simulink model "conveyor_belt_system_models_in_simulink"  (R2023a)
settings: Solver=VariableStepAuto  StartTime=0.0  StopTime=120  RelTol=1e-3
undefined symbols (not defined in the file): b, Fv, G, J, K1, K2, K3, Kphi, L, Mc, R, R_pully
libraries: slpidlib x1
settings Model: Creator=ARABI  LastModifiedBy=ARABI

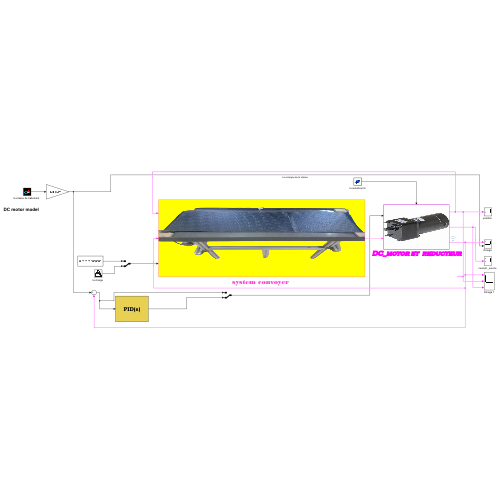
[thumbnail: Simulink's stored preview of the top-level diagram]
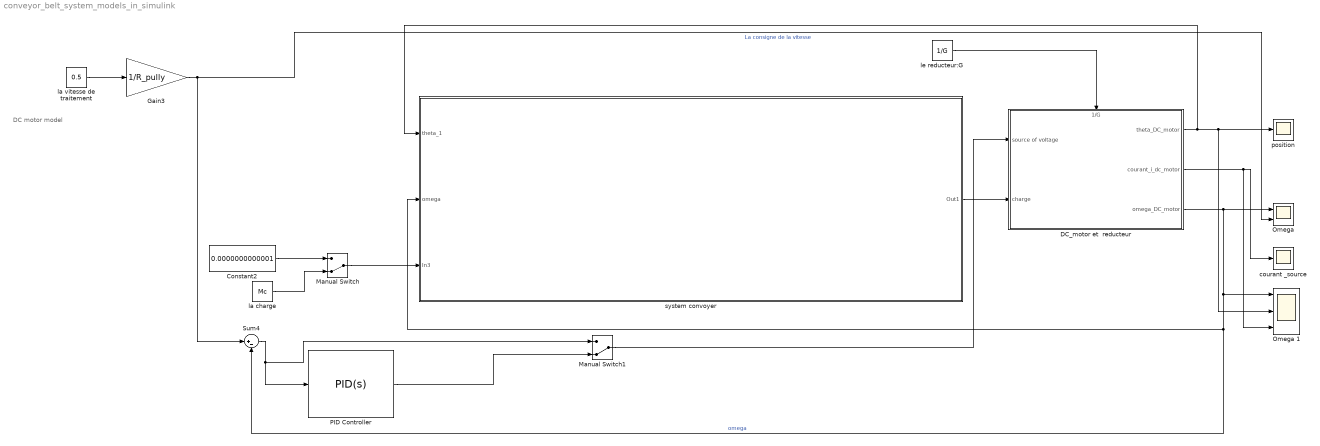
== system conveyor_belt_system_models_in_simulink ==
  note: DC motor model
  Constant2 : Constant  Value=0.0000000000001
  DC_motor et  reducteur : Subsystem
      settings: PortSchema="{\"entries\":[{\"content\":{\"sides\":[{\"content\":{\"connectorIds\":[\"In1\",\"In2\"]},\"type\":\"ConnectorPlacement.EquallySpacedRectSide\",\"uuid\":\"26fbfc1a-56c7-4e56-9ac7-29104c9994d4\"},{\"content\":{\"connectorIds\":[\"Out1\",\"Out2\",\"Out3\"],\"side\":\"RIGHT\"},\"type\":\"ConnectorPlacement.EquallySpacedRectSide\",\"uuid\":\"e16094de-f307-4a64-93f4-279fc46fd241\"},{\"content\":{\"connectorIds\":[\"In3\"],\"side\":\"TOP\"},\"type\":\"ConnectorPlacement.EquallySpacedRectSide\",\"uuid\":\"6a3015f2-a4f9-4d11-9390-c80012a11723\"}]},\"type\":\"ConnectorPlacement.EquallySpacedConnector\",\"uuid\":\"83312b76-c8d9-4603-a222-ebea70a19c3f\"}],\"packageUris\":[\"http://schema.mathworks.com/mf0/Connector/R2020b\"],\"version\":\"1.0\"}"
      mask Display: image('OIP.jpeg'); % Use "Edit Image" on toolstrip to change.
  Gain3 : Gain  Gain=1/R_pully
  Manual Switch : ManualSwitch  CurrentSetting=0
  Manual Switch1 : ManualSwitch  CurrentSetting=0
  "Omega " : Scope  NumInputPorts=2
  Omega 1 : Scope  NumInputPorts=3
  PID Controller : slpidlib/PID Controller  Controller=PID  Form=Parallel  TimeDomain=Continuous-time  UseExternalTs=off  SampleTime=-1  IntegratorMethod=Forward Euler  FilterMethod=Forward Euler  ControllerParametersSource=internal  P=1  I=1  UseKiTs=off  D=0  N=100  UseFilter=on  TunerSelectOption=Transfer Function Based (PID Tuner App)  InitialConditionSource=internal  InitialConditionForIntegrator=0  InitialConditionForFilter=0  DifferentiatorICPrevScaledInput=0  ExternalReset=none  TrackingMode=off  Kt=1  LimitOutput=off  SatLimitsSource=internal  UpperSaturationLimit=inf  LowerSaturationLimit=-inf  LinearizeAsGain=on  AntiWindupMode=none  Kb=1  LimitIntegrator=off  UpperIntegratorSaturationLimit=inf  LowerIntegratorSaturationLimit=-inf  POutMin=[]  POutMax=[]  IOutMin=[]  IOutMax=[]  DOutMin=[]  DOutMax=[]  NOutMin=[]  NOutMax=[]  SumOutMin=[]  SumOutMax=[]  SaturationOutMin=[]  SaturationOutMax=[]  PParamMin=[]  PParamMax=[]  IParamMin=[]  IParamMax=[]  DParamMin=[]  DParamMax=[]  NParamMin=[]  NParamMax=[]  KbParamMin=[]  KbParamMax=[]  KtParamMin=[]  KtParamMax=[]  KbOutMin=[]  KbOutMax=[]  KtOutMin=[]  KtOutMax=[]  IntegratorOutMin=[]  IntegratorOutMax=[]  FilterOutMin=[]  FilterOutMax=[]  SumI1OutMin=[]  SumI1OutMax=[]  SumI2OutMin=[]  SumI2OutMax=[]  SumI3OutMin=[]  SumI3OutMax=[]  SumI4OutMin=[]  SumI4OutMax=[]  SumDOutMin=[]  SumDOutMax=[]  DifferentiatorOutMin=[]  DifferentiatorOutMax=[]  FilterDiffOutCoefMin=[]  FilterDiffOutCoefMax=[]  ReciprocalOutMin=[]  ReciprocalOutMax=[]  SumDenOutMin=[]  SumDenOutMax=[]  SumNumOutMin=[]  SumNumOutMax=[]  DivideOutMin=[]  DivideOutMax=[]  UdiffTsProdOutMin=[]  UdiffTsProdOutMax=[]  NTsProdOutMin=[]  NTsProdOutMax=[]  UintegralTsProdOutMin=[]  UintegralTsProdOutMax=[]  UngainTsProdOutMin=[]  UngainTsProdOutMax=[]  ClampingZeroOutDataTypeStr=Inherit: Inherit via back propagation  ClampingZeroOutMin=[]  ClampingZeroOutMax=[]  FilterDenConstantOutDataTypeStr=Inherit: Inherit via back propagation  FilterDenConstantOutMin=[]  FilterDenConstantOutMax=[]  PCopyOutDataTypeStr=Inherit: Inherit via back propagation  PCopyOutMin=[]  PCopyOutMax=[]  NCopyOutDataTypeStr=Inherit: Inherit via back propagation  NCopyOutMin=[]  NCopyOutMax=[]  IntegratorContinuousStateAttributes=''  IntegratorStateMustResolveToSignalObject=off  IntegratorRTWStateStorageClass=Auto  FilterContinuousStateAttributes=''  FilterStateMustResolveToSignalObject=off  FilterRTWStateStorageClass=Auto  ParallelPVariant=InternalParameters  IdealPVariant=Disabled  IVariant=InternalParameters  DVariant=InternalParameters  IntegratorVariant=Continuous  SatVariant=Disabled  AWVariant=Passthrough  PCopyVariant=Disabled  TRVariant=Disabled  FdbkBlocksVariant=Forward  IdealPFdbkVariant=Disabled  SatFdbkVariant=Disabled  DerivativeFilterVariant=ContFilter  NVariant=InternalParameters  NCopyVariant=Disabled  FilterICVariant=InternalICsFilter  IntegratorICVariant=InternalICs  ExternalResetVariant=Disabled  TRSumVariant=Passthrough  SumFdbkVariant=Disabled  SumVariant=Sum_PID  TsampFilterVariant=InternalTs  TsampNgainVariant=Passthrough  TsampIntegralVariant=Disabled_SignalSpec  ExternalSaturationOutDataTypeStr=Inherit: Same as second input
  Sum4 : Sum  Inputs=|+-
  "courant _source " : Scope
  "la charge " : Constant  Value=Mc
      mask Display: image('download (1).jpeg'); % Use "Edit Image" on toolstrip to change.
  "la vitesse de traitement  " : Constant  Value=0.5
      mask Display: image('download.jpeg'); % Use "Edit Image" on toolstrip to change.
  le reducteur:G : Constant  Value=1/G
      mask Display: image('Reductor-pendular-rossi.jpg'); % Use "Edit Image" on toolstrip to change.
  "position " : Scope
  "system convoyer " : Subsystem
      mask Display: image('$imagefile'); % Use "Edit Image" on toolstrip to change.
  wires:
  le reducteur:G/1 -> DC_motor et  reducteur/3(1/G)
  "la vitesse de traitement  "/1 -> Gain3/1
  Gain3/1 -> Sum4/1, "Omega "/2  "La consigne de la vitesse"
  "la charge "/1 -> Manual Switch/2
  Manual Switch/1 -> "system convoyer "/3(In3)
  Constant2/1 -> Manual Switch/1
  PID Controller/1 -> Manual Switch1/2
  Sum4/1 -> PID Controller/1, Manual Switch1/1
  "system convoyer "/1(Out1) -> DC_motor et  reducteur/2("charge ")
  Manual Switch1/1 -> DC_motor et  reducteur/1("source of voltage ")
  DC_motor et  reducteur/1(theta_DC_motor) -> "position "/1, Omega 1/2, "system convoyer "/1(theta_1)
  DC_motor et  reducteur/2(courant_i_dc_motor) -> Omega 1/3, "courant _source "/1
  DC_motor et  reducteur/3(omega_DC_motor) -> Sum4/2, "system convoyer "/2(omega), Omega 1/1, "Omega "/1  "omega"

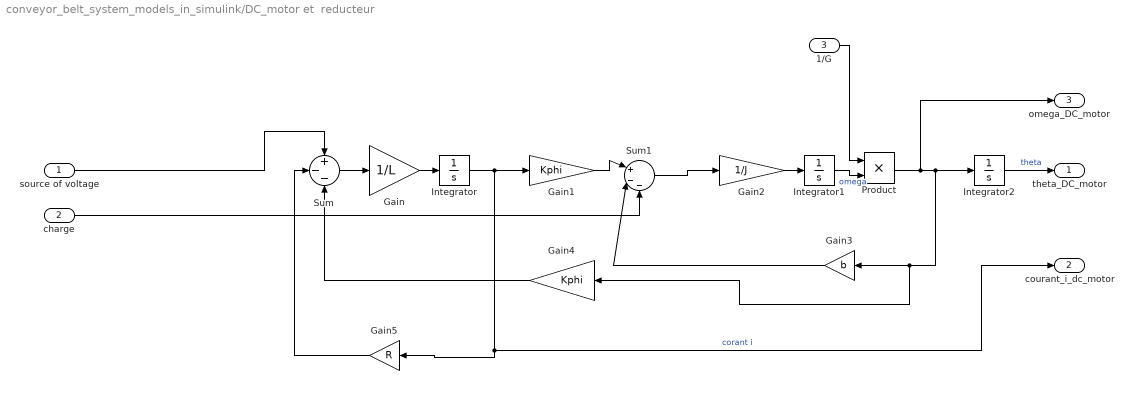
== system conveyor_belt_system_models_in_simulink/DC_motor et  reducteur ==
  "source of voltage " : Inport
  "charge " : Inport  Port=2
  1/G : Inport  Port=3
  Gain : Gain  Gain=1/L
  Gain1 : Gain  Gain=Kphi
  Gain2 : Gain  Gain=1/J
  Gain3 : Gain  Gain=b
  Gain4 : Gain  Gain=Kphi
  Gain5 : Gain  Gain=R
  Integrator : Integrator
  Integrator1 : Integrator
  Integrator2 : Integrator
  Product : Product
  Sum : Sum  Inputs=+--
  Sum1 : Sum  Inputs=|+--
  theta_DC_motor : Outport
  courant_i_dc_motor : Outport  Port=2
  omega_DC_motor : Outport  Port=3
  wires:
  "source of voltage "/1 -> Sum/1
  Sum/1 -> Gain/1
  Gain/1 -> Integrator/1
  Integrator/1 -> Gain5/1, courant_i_dc_motor/1, Gain1/1  "corant i"
  Gain1/1 -> Sum1/1
  Sum1/1 -> Gain2/1
  Gain2/1 -> Integrator1/1
  Integrator1/1 -> Product/2  "omega"
  Gain3/1 -> Sum1/2
  Gain4/1 -> Sum/3
  Gain5/1 -> Sum/2
  Integrator2/1 -> theta_DC_motor/1  "theta"
  "charge "/1 -> Sum1/3
  Product/1 -> omega_DC_motor/1, Integrator2/1, Gain4/1, Gain3/1
  1/G/1 -> Product/1

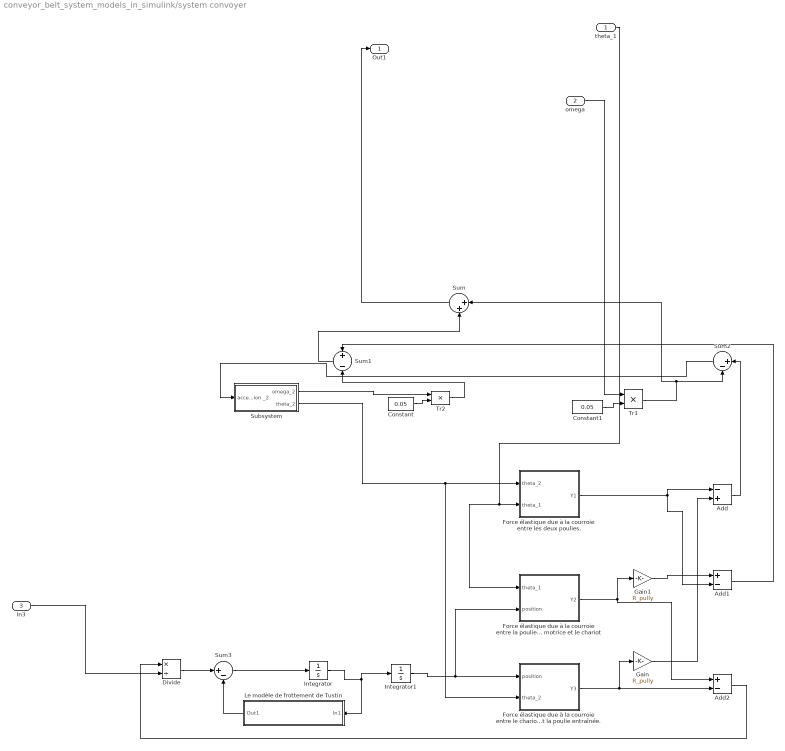
== system conveyor_belt_system_models_in_simulink/system convoyer  ==
  theta_1 : Inport
  omega : Inport  Port=2
  In3 : Inport  Port=3
  Add : Sum  Inputs=-+
  Add1 : Sum  Inputs=+-
  Add2 : Sum  Inputs=+-
  Constant : Constant  Value=0.05
  Constant1 : Constant  Value=0.05
  Divide : Product  Inputs=*/
  Force élastique due à la courroie entre la poulie motrice et le chariot : Subsystem
  Force élastique due à la courroie entre le chariot et la poulie entraînée. : Subsystem
  Force élastique due à la courroie entre les deux poulies. : Subsystem
  Gain : Gain  Gain=R_pully
  Gain1 : Gain  Gain=R_pully
  Integrator : Integrator
  Integrator1 : Integrator
  "Le modèle de frottement de Tustin " : Subsystem
  Subsystem : Subsystem
  Sum : Sum  Inputs=|++
  Sum1 : Sum  Inputs=+-
  Sum2 : Sum  Inputs=|+-
  Sum3 : Sum  Inputs=|+-
  Tr1 : Product
  Tr2 : Product
  Out1 : Outport
  wires:
  "Le modèle de frottement de Tustin "/1(Out1) -> Sum3/2
  theta_1/1 -> Force élastique due à la courroie entre la poulie motrice et le chariot/1(theta_1), Force élastique due à la courroie entre les deux poulies./2(theta_1)
  Force élastique due à la courroie entre le chariot et la poulie entraînée./1(Y3) -> Gain/1, Add2/2
  Sum2/1 -> Subsystem/1(acceliration _2)
  Subsystem/1(omega_2) -> Tr2/1
  Integrator/1 -> "Le modèle de frottement de Tustin "/1(In1), Integrator1/1
  Sum/1 -> Out1/1
  Integrator1/1 -> Force élastique due à la courroie entre le chariot et la poulie entraînée./1(position), Force élastique due à la courroie entre la poulie motrice et le chariot/2(position)
  Tr1/1 -> Sum2/2, Sum/1
  Constant1/1 -> Tr1/2
  Sum3/1 -> Integrator/1
  Divide/1 -> Sum3/1
  Subsystem/2(theta_2) -> Force élastique due à la courroie entre les deux poulies./1(theta_2), Force élastique due à la courroie entre le chariot et la poulie entraînée./2(theta_2)
  Add2/1 -> Divide/1
  Tr2/1 -> Sum1/2
  In3/1 -> Divide/2
  Add1/1 -> Sum1/1
  Add/1 -> Sum2/1
  Gain1/1 -> Add1/1
  Gain/1 -> Add/2
  Sum1/1 -> Sum/2
  Force élastique due à la courroie entre la poulie motrice et le chariot/1(Y2) -> Add2/1, Gain1/1
  Force élastique due à la courroie entre les deux poulies./1(Y1) -> Add1/2, Add/1
  Constant/1 -> Tr2/2
  omega/1 -> Tr1/1

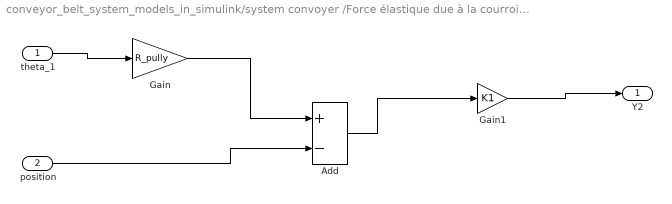
== system conveyor_belt_system_models_in_simulink/system convoyer /Force élastique due à la courroie entre la poulie motrice et le chariot ==
  theta_1 : Inport
  position : Inport  Port=2
  Add : Sum  Inputs=+-
  Gain : Gain  Gain=R_pully
  Gain1 : Gain  Gain=K1
  Y2 : Outport
  wires:
  theta_1/1 -> Gain/1
  position/1 -> Add/2
  Gain/1 -> Add/1
  Add/1 -> Gain1/1
  Gain1/1 -> Y2/1

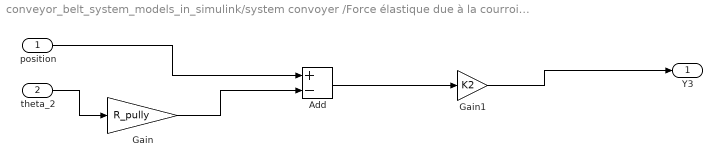
== system conveyor_belt_system_models_in_simulink/system convoyer /Force élastique due à la courroie entre le chariot et la poulie entraînée. ==
  position : Inport
  theta_2 : Inport  Port=2
  Add : Sum  Inputs=+-
  Gain : Gain  Gain=R_pully
  Gain1 : Gain  Gain=K2
  Y3 : Outport
  wires:
  Add/1 -> Gain1/1
  position/1 -> Add/1
  theta_2/1 -> Gain/1
  Gain/1 -> Add/2
  Gain1/1 -> Y3/1

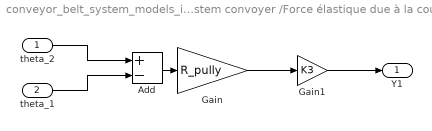
== system conveyor_belt_system_models_in_simulink/system convoyer /Force élastique due à la courroie entre les deux poulies. ==
  theta_2 : Inport
  theta_1 : Inport  Port=2
  Add : Sum  Inputs=+-
  Gain : Gain  Gain=R_pully
  Gain1 : Gain  Gain=K3
  Y1 : Outport
  wires:
  theta_2/1 -> Add/1
  theta_1/1 -> Add/2
  Add/1 -> Gain/1
  Gain/1 -> Gain1/1
  Gain1/1 -> Y1/1

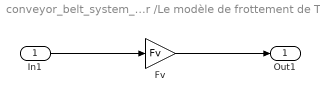
== system conveyor_belt_system_models_in_simulink/system convoyer /Le modèle de frottement de Tustin  ==
  In1 : Inport
  Fv : Gain  Gain=Fv
  Out1 : Outport
  wires:
  In1/1 -> Fv/1
  Fv/1 -> Out1/1

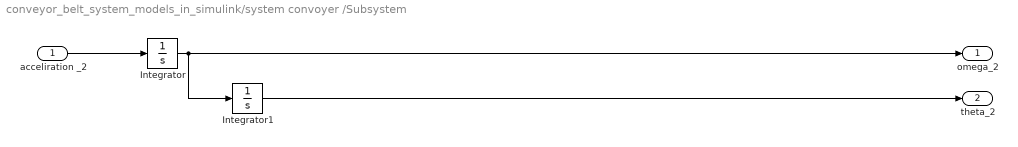
== system conveyor_belt_system_models_in_simulink/system convoyer /Subsystem ==
  acceliration _2 : Inport
  Integrator : Integrator
  Integrator1 : Integrator
  omega_2 : Outport
  theta_2 : Outport  Port=2
  wires:
  acceliration _2/1 -> Integrator/1
  Integrator/1 -> omega_2/1, Integrator1/1
  Integrator1/1 -> theta_2/1
